simulink model "simpleRC"  (R2023b)
settings: Solver=VariableStepAuto  StartTime=0.0  StopTime=10  RelTol=1e-3
values from neighbouring files (symbols this model uses):
  C = 1e-6    (= 1e-06)    [RC_P2.m]
  R = 1000    [RC_P2.m]
settings Model: Creator=ascom  LastModifiedBy=ascom

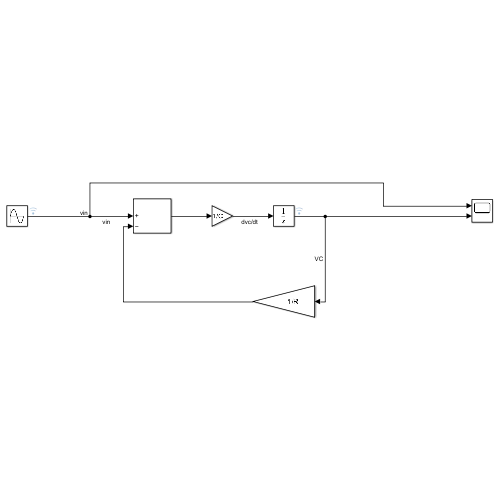
[thumbnail: Simulink's stored preview of the top-level diagram]
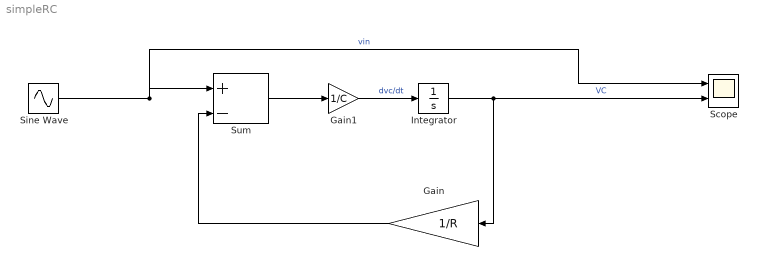
== system simpleRC ==
  Gain : Gain  Gain=1/R
  Gain1 : Gain  Gain=1/C
  Integrator : Integrator
  Scope : Scope  NumInputPorts=2
  Sine Wave : Sin  Amplitude=5  SampleTime=0
  Sum : Sum  Inputs=|+-
  wires:
  Sine Wave/1 -> Scope/1, Sum/1  "vin"
  Sum/1 -> Gain1/1
  Gain/1 -> Sum/2
  Gain1/1 -> Integrator/1  "dvc/dt"
  Integrator/1 -> Gain/1, Scope/2  "VC"
